simulink model "Test_PIL_IIR_Filter"  (R2018b)
settings: configuration reference "Test_PIL_IIR_Filter_config_ref" (kept outside this file)
PreLoadFcn:
  | run iir_startup;
  | load('Test_PIL_IIR_Filter_config_ref.mat');
model workspace (MAT data in the model file):
  dataint = Simulink.Signal
  dataint.DataType = 'int32'
  dataint.Dimensions = -1
  dataint.DimensionsMode = 'auto'
  dataint.Complexity = 'real'
  dataint.SampleTime = -1
  dataint.SamplingMode = 'auto'
  dataint.InitialValue = '0'
libraries: simulink x1
CloseFcn:
  | clear Test_PIL_IIR_Filter_config_ref;
  | clear a1;
  | clear b0;
  | clear t;
  | clear testdata;
settings Model: DataTypeOverrideAppliesTo=Floating-point  Creator=obas  LastModifiedBy=fenard1
settings ConfigSetRef: SourceLocation=Base Workspace

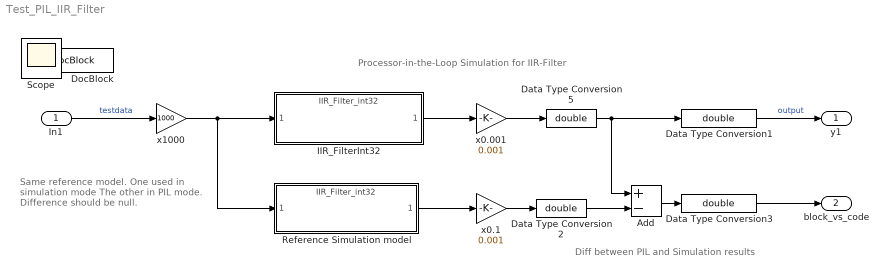
== system Test_PIL_IIR_Filter ==
  note: Same reference model.
      | One used in simulation mode
      | The other in PIL mode.
      | Difference should be null.
  note: Diff between PIL and Simulation results
  note: Processor-in-the-Loop Simulation for IIR-Filter
  In1 : Inport  OutDataTypeStr=double  PortDimensions=1  SampleTime=0.001  Interpolate=off
  Add : Sum  Inputs=+-
  Data Type Conversion{1..3,5} (4 alike) : DataTypeConversion  OutDataTypeStr=double  SaturateOnIntegerOverflow=on  RndMeth=Zero
  DocBlock : simulink/Model-Wide Utilities/DocBlock  DocumentType=Text
      content=|
      | The model contains a 1st-order IIR filter of the following form:
      |
      |     y(n) = a1*y(n-1) + b0*u(n)
      |
      | Using the model pre-load function callback:
      |
      |     a1 = 0.9
      |     b0 = 0.1
      |
      | The filter is sampled at 1000Hz.
      |
      | Modified from iir_filter.mdl to enable ERT code generation.
  IIR_FilterInt32 : ModelReference  ModelNameDialog=IIR_Filter_int32.slx  SimulationMode=Processor-in-the-loop (PIL)  ModelReferenceVersion=1.115
  Reference Simulation model : ModelReference  ModelNameDialog=IIR_Filter_int32.slx  SimulationMode=Normal  ModelReferenceVersion=1.115
  x0.001 : Gain  Gain=0.001
  x0.1 : Gain  Gain=0.001
  x1000 : Gain  Gain=1000  ParamDataTypeStr=uint32  OutMin=-2147483647-1  OutMax=2147483647  OutDataTypeStr=int32
  y1 : Outport
  block_vs_code : Outport  Port=2
  Scope : Scope
  wires:
  In1/1 -> x1000/1  "testdata"
  Data Type Conversion1/1 -> y1/1  "output"
  Data Type Conversion3/1 -> block_vs_code/1
  Add/1 -> Data Type Conversion3/1
  Data Type Conversion5/1 -> Add/1, Data Type Conversion1/1
  x0.001/1 -> Data Type Conversion5/1
  x1000/1 -> Reference Simulation model/1, IIR_FilterInt32/1
  IIR_FilterInt32/1 -> x0.001/1
  x0.1/1 -> Data Type Conversion2/1
  Reference Simulation model/1 -> x0.1/1
  Data Type Conversion2/1 -> Add/2
